simulink model "model_simulation"  (R2024a)
settings: Solver=ode4  StartTime=0.0  StopTime=2  FixedStep=0.0001  RelTol=1e-3
values from neighbouring files (symbols this model uses):
  c = 0.5    [parameters.m]
  d = 0.5    [parameters.m]
  eta = 0.9    [parameters.m]
  init_angles = [0;0;2/180*pi]    [main.m]
  init_dangles = [0;0;0]    [main.m]
  Km = 0.05    [parameters.m]
  L = 2.6e-3    (= 0.0026)    [parameters.m]    (also in pole_placement_Luenberger.m = place(A', C', desired_poles)')
  N = 50    [parameters.m]
  r = 0.044    [parameters.m]
  R = 0.5    [parameters.m]
undefined symbols (not defined in the file or in its folder): tau_m
libraries: slpidlib x1
settings Model: Creator=albin  LastModifiedBy=albin
settings DataIOCC: ExternalInput=[t, 0, 0]

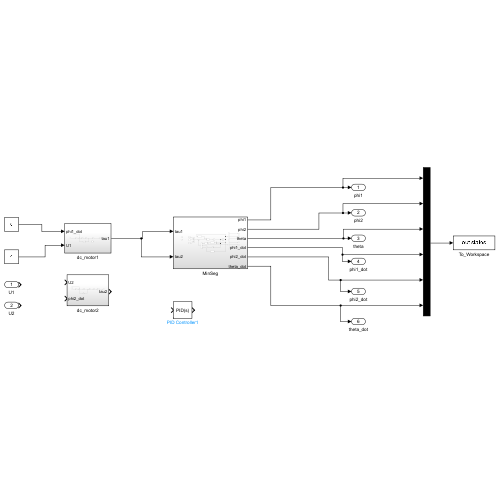
[thumbnail: Simulink's stored preview of the top-level diagram]
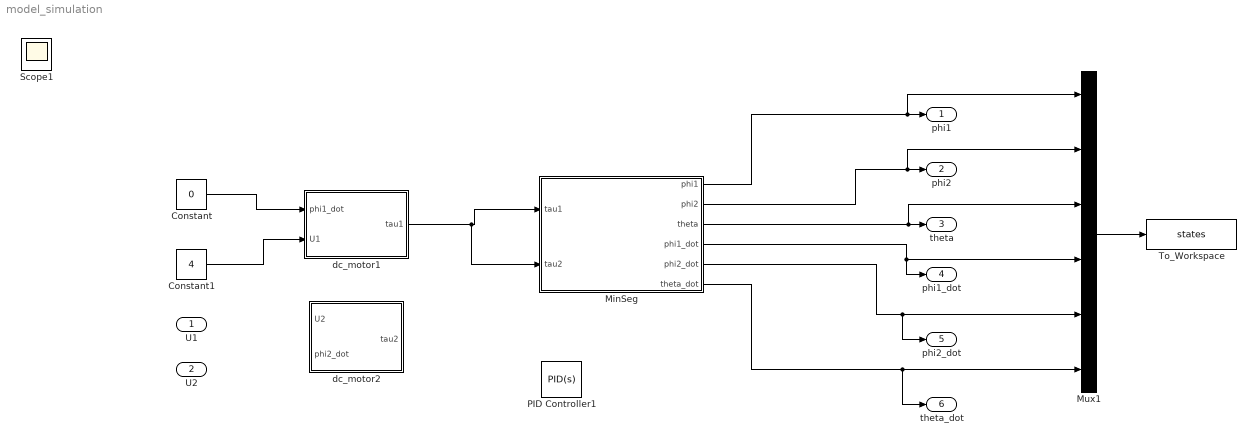
== system model_simulation ==
  U1 : Inport
  U2 : Inport  Port=2
  Constant : Constant  Value=0
  Constant1 : Constant  Value=4
  MinSeg : Subsystem
  Mux1 : Mux  Inputs=6
  PID Controller1 : slpidlib/PID Controller  Controller=PID  Form=Parallel  TimeDomain=Continuous-time  UseExternalTs=off  SampleTime=-1  IntegratorMethod=Forward Euler  FilterMethod=Forward Euler  ControllerParametersSource=internal  P=-0.117345401430051  I=-0.52973367050469  UseKiTs=off  D=-0.00496147609503641  UseExternalDerivativeSource=off  N=145.579587440428  UseFilter=on  TunerSelectOption=Transfer Function Based (PID Tuner App)  InitialConditionSource=internal  InitialConditionForIntegrator=0  InitialConditionForFilter=0  DifferentiatorICPrevScaledInput=0  ExternalReset=none  TrackingMode=off  Kt=1  LimitOutput=off  SatLimitsSource=internal  UpperSaturationLimit=inf  LowerSaturationLimit=-inf  LinearizeAsGain=on  AntiWindupMode=none  Kb=1  LimitIntegrator=off  UpperIntegratorSaturationLimit=inf  LowerIntegratorSaturationLimit=-inf  POutMin=[]  POutMax=[]  IOutMin=[]  IOutMax=[]  DOutMin=[]  DOutMax=[]  NOutMin=[]  NOutMax=[]  SumOutMin=[]  SumOutMax=[]  SaturationOutMin=[]  SaturationOutMax=[]  PParamMin=[]  PParamMax=[]  IParamMin=[]  IParamMax=[]  DParamMin=[]  DParamMax=[]  NParamMin=[]  NParamMax=[]  KbParamMin=[]  KbParamMax=[]  KtParamMin=[]  KtParamMax=[]  KbOutMin=[]  KbOutMax=[]  KtOutMin=[]  KtOutMax=[]  IntegratorOutMin=[]  IntegratorOutMax=[]  FilterOutMin=[]  FilterOutMax=[]  SumI1OutMin=[]  SumI1OutMax=[]  SumI2OutMin=[]  SumI2OutMax=[]  SumI3OutMin=[]  SumI3OutMax=[]  SumI4OutMin=[]  SumI4OutMax=[]  SumDOutMin=[]  SumDOutMax=[]  DifferentiatorOutMin=[]  DifferentiatorOutMax=[]  FilterDiffOutCoefMin=[]  FilterDiffOutCoefMax=[]  ReciprocalOutMin=[]  ReciprocalOutMax=[]  SumDenOutMin=[]  SumDenOutMax=[]  SumNumOutMin=[]  SumNumOutMax=[]  DivideOutMin=[]  DivideOutMax=[]  UdiffTsProdOutMin=[]  UdiffTsProdOutMax=[]  NTsProdOutMin=[]  NTsProdOutMax=[]  UintegralTsProdOutMin=[]  UintegralTsProdOutMax=[]  UngainTsProdOutMin=[]  UngainTsProdOutMax=[]  ClampingZeroOutDataTypeStr=Inherit: Inherit via back propagation  ClampingZeroOutMin=[]  ClampingZeroOutMax=[]  FilterDenConstantOutDataTypeStr=Inherit: Inherit via back propagation  FilterDenConstantOutMin=[]  FilterDenConstantOutMax=[]  PCopyOutDataTypeStr=Inherit: Inherit via back propagation  PCopyOutMin=[]  PCopyOutMax=[]  NCopyOutDataTypeStr=Inherit: Inherit via back propagation  NCopyOutMin=[]  NCopyOutMax=[]  IntegratorContinuousStateAttributes=''  IntegratorStateMustResolveToSignalObject=off  IntegratorRTWStateStorageClass=Auto  FilterContinuousStateAttributes=''  FilterStateMustResolveToSignalObject=off  FilterRTWStateStorageClass=Auto  ParallelPVariant=InternalParameters  IdealPVariant=Disabled  IVariant=InternalParameters  DVariant=InternalParameters  IntegratorVariant=Continuous  SatVariant=Disabled  AWVariant=Passthrough  PCopyVariant=Disabled  TRVariant=Disabled  FdbkBlocksVariant=Forward  IdealPFdbkVariant=Disabled  SatFdbkVariant=Disabled  DerivativeFilterVariant=ContFilter  NVariant=InternalParameters  NCopyVariant=Disabled  FilterICVariant=InternalICsFilter  IntegratorICVariant=InternalICs  ExternalResetVariant=Disabled  TRSumVariant=Passthrough  SumFdbkVariant=Disabled  SumVariant=Sum_PID  TsampFilterVariant=InternalTs  TsampNgainVariant=Passthrough  TsampIntegralVariant=Disabled_SignalSpec  ExternalSaturationOutDataTypeStr=Inherit: Same as second input  DerivativeSourceVariant=ErrorSignal
  To_Workspace : ToWorkspace  VariableName=states  SaveFormat=Timeseries  SampleTime=-1
  dc_motor1 : Subsystem
  dc_motor2 : Subsystem
  phi1 : Outport
  phi2 : Outport  Port=2
  theta : Outport  Port=3
  phi1_dot : Outport  Port=4
  phi2_dot : Outport  Port=5
  theta_dot : Outport  Port=6
  Scope1 : Scope
  wires:
  Mux1/1 -> To_Workspace/1
  MinSeg/1(phi1) -> Mux1/1, phi1/1
  MinSeg/2(phi2) -> Mux1/2, phi2/1
  MinSeg/3(theta) -> Mux1/3, theta/1
  MinSeg/4(phi1_dot) -> phi1_dot/1, Mux1/4
  MinSeg/5(phi2_dot) -> phi2_dot/1, Mux1/5
  MinSeg/6(theta_dot) -> Mux1/6, theta_dot/1
  Constant/1 -> dc_motor1/1(phi1_dot)
  Constant1/1 -> dc_motor1/2(U1)
  dc_motor1/1(tau1) -> MinSeg/2(tau2), MinSeg/1(tau1)

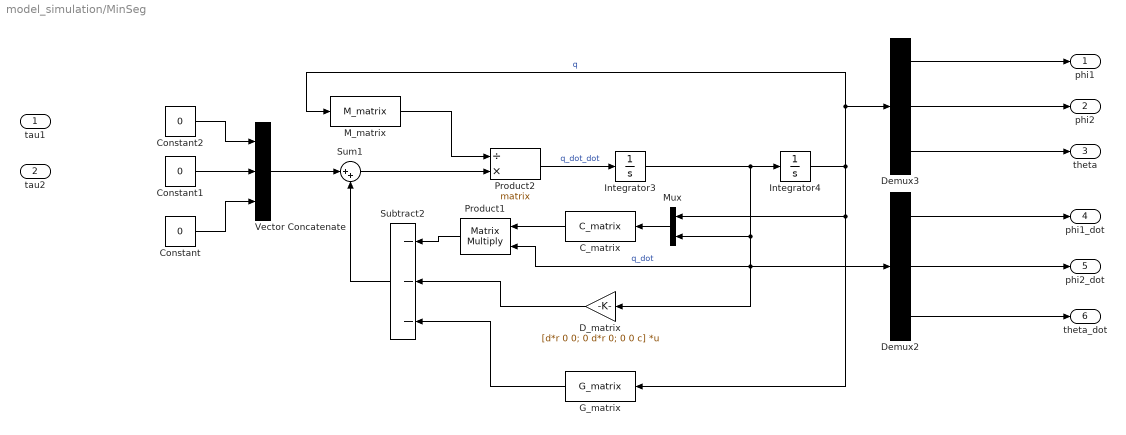
== system model_simulation/MinSeg ==
  tau1 : Inport
  tau2 : Inport  Port=2
  C_matrix : MATLABFcn  MATLABFcn=C_matrix  OutputDimensions=[3,3]  Output1D=off
  Constant : Constant  Value=0
  Constant1 : Constant  Value=0
  Constant2 : Constant  Value=0
  D_matrix : Gain  Gain=[d*r 0 0; 0 d*r 0; 0 0 c]  Multiplication=Matrix(K*u)
  Demux2 : Demux  Outputs=3
  Demux3 : Demux  Outputs=3
  G_matrix : MATLABFcn  MATLABFcn=G_matrix  OutputDimensions=[3,1]  Output1D=off
  Integrator3 : Integrator  InitialCondition=init_dangles
  Integrator4 : Integrator  InitialCondition=init_angles
  M_matrix : MATLABFcn  MATLABFcn=M_matrix  OutputDimensions=[3,3]  Output1D=off
  Mux : Mux  Inputs=2
  Product1 : Product  Multiplication=Matrix(*)
  Product2 : Product  Inputs=/*  Multiplication=Matrix(*)
  Subtract2 : Sum  Inputs=---
  Sum1 : Sum  Inputs=|++
  Vector Concatenate : Concatenate  NumInputs=3
  phi1 : Outport
  phi2 : Outport  Port=2
  theta : Outport  Port=3
  phi1_dot : Outport  Port=4
  phi2_dot : Outport  Port=5
  theta_dot : Outport  Port=6
  wires:
  Product2/1 -> Integrator3/1  "q_dot_dot"
  Vector Concatenate/1 -> Sum1/1
  Constant/1 -> Vector Concatenate/3
  Mux/1 -> C_matrix/1
  Integrator4/1 -> G_matrix/1, Mux/1, M_matrix/1, Demux3/1  "q"
  Demux3/2 -> phi2/1
  Demux2/1 -> phi1_dot/1
  M_matrix/1 -> Product2/1
  Demux3/1 -> phi1/1
  Integrator3/1 -> D_matrix/1, Product1/2, Demux2/1, Mux/2, Integrator4/1  "q_dot"
  G_matrix/1 -> Subtract2/3
  Subtract2/1 -> Sum1/2
  C_matrix/1 -> Product1/1
  Product1/1 -> Subtract2/1
  Constant1/1 -> Vector Concatenate/2
  Demux2/3 -> theta_dot/1
  Demux2/2 -> phi2_dot/1
  Demux3/3 -> theta/1
  Sum1/1 -> Product2/2
  Constant2/1 -> Vector Concatenate/1
  D_matrix/1 -> Subtract2/2

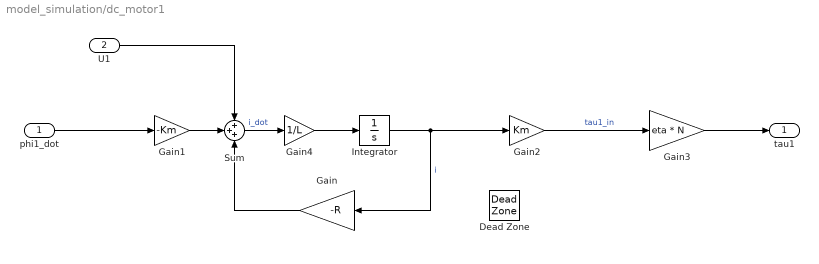
== system model_simulation/dc_motor1 ==
  phi1_dot : Inport
  U1 : Inport  Port=2
  Dead Zone : DeadZone  LowerValue=-tau_m  UpperValue=tau_m
  Gain : Gain  Gain=-R
  Gain1 : Gain  Gain=-Km
  Gain2 : Gain  Gain=Km
  Gain3 : Gain  Gain=eta * N
  Gain4 : Gain  Gain=1/L
  Integrator : Integrator
  Sum : Sum  Inputs=+++
  tau1 : Outport
  wires:
  Gain2/1 -> Gain3/1  "tau1_in"
  Integrator/1 -> Gain/1, Gain2/1  "i"
  Gain3/1 -> tau1/1
  Gain1/1 -> Sum/2
  Gain/1 -> Sum/3
  phi1_dot/1 -> Gain1/1
  Sum/1 -> Gain4/1  "i_dot"
  Gain4/1 -> Integrator/1
  U1/1 -> Sum/1

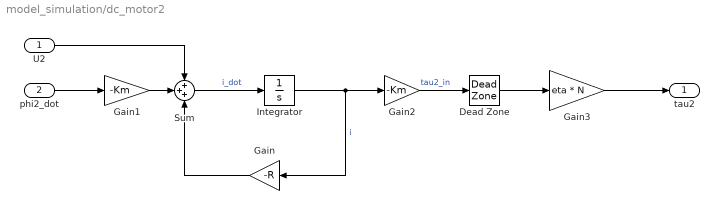
== system model_simulation/dc_motor2 ==
  U2 : Inport
  phi2_dot : Inport  Port=2
  Dead Zone : DeadZone  LowerValue=-0.005  UpperValue=0.005
  Gain : Gain  Gain=-R
  Gain1 : Gain  Gain=-Km
  Gain2 : Gain  Gain=-Km
  Gain3 : Gain  Gain=eta * N
  Integrator : Integrator
  Sum : Sum  Inputs=+++
  tau2 : Outport
  wires:
  Gain2/1 -> Dead Zone/1  "tau2_in"
  Integrator/1 -> Gain/1, Gain2/1  "i"
  Gain3/1 -> tau2/1
  U2/1 -> Sum/1
  Gain1/1 -> Sum/2
  Sum/1 -> Integrator/1  "i_dot"
  phi2_dot/1 -> Gain1/1
  Gain/1 -> Sum/3
  Dead Zone/1 -> Gain3/1
